simulink model "d_motor"  (Simulink 5.1)
settings: Solver=ode45  StartTime=0.0  StopTime=10.0  RelTol=1e-3
settings Model: Creator=fmilano  LastModifiedBy=fmilano  SignalLoggingName=logsout  BooleanDataType=on  RTWOptions="-aEnforceIntegerDowncast=1 -aFoldNonRolledExpr=1 -aInlineInvariantSignals=0 -aInlineParameters=0 -aLocalBlockOutputs=1 -aRollThreshold=5 -aZeroInternalMemoryAtStartup=1 -aZeroExternalMemoryAtStartup=1 -aInitFltsAndDblsToZero=0 -aForceBlockIOInitOptimize=0 -aGenerateReport=0 -aGenCodeOnly=0 -aRTWVerbose=1 -aIncludeHyperlinkInReport=0 -aLaunchReport=0 -aGenerateTraceInfo=0  -aForceParamTrailComments=0 -aGenerateComments=1 -aIgnoreCustomStorageClasses=1 -aIncHierarchyInIds=0 -aMaxRTWIdLen=31 -aShowEliminatedStatements=0 -aIncDataTypeInIds=0 -aInsertBlockDesc=0 -aIgnoreTestpoints=0 -aSimulinkBlockComments=1 -aInlinedPrmAccess=\"Literals\"  -aSuppressErrorStatus=0 -aModelReferenceCompliant=1 -aParenthesesLevel=\"Nominal\" -aModelStepFunctionPrototypeControlCompliant=0 -aPortableWordSizes=0 -aParMdlRefBuildCompliant=1 -aSupportNonInlinedSFcns=1 -aSupportContinuousTime=1 -aSupportComplex=1 -aSupportNonFinite=1 -aSupportAbsoluteTime=1 -aMultiwordLength=2048 -aTargetPreCompLibLocation=\"\" -aTargetLibSuffix=\"\" -aTargetFunctionLibrary=\"ANSI_C\" -aTargetFcnLib=\"ansi_tfl_tmw.mat\" -aMultiInstanceERTCode=0 -aLogVarNameModifier=\"rt_\" -aERTFirstTimeCompliant=0 -aIsPILTarget=0 -aCombineOutputUpdateFcns=0 -aGenerateASAP2=0 -aGenerateClassInterface=0 -aGenerateTestInterfaces=0 -aGenerateSampleERTMain=0 -aGenerateFullHeader=1 -aUtilityFuncGeneration=\"Auto\" -aIncludeFileDelimiter=\"Auto\" -aIncludeMdlTerminateFcn=1 -aPurelyIntegerCode=0 -aAutosarCompliant=0 -aERTCustomFileBanners=0 -aRTWCAPIStates=0 -aRTWCAPIParams=0 -aRTWCAPISignals=0 -aMatFileLogging=1 -aCompOptLevelCompliant=1 -aCPPClassGenCompliant=0 -aExtModeIntrfLevel=\"Level1\" -aExtModeMexFile=\"ext_comm\" -aExtModeTransport=0 -aExtModeStaticAllocSize=1000000 -aExtModeTesting=0 -aExtModeStaticAlloc=0 -aExtMode=0 -aERTMultiwordLength=256 -aERTMultiwordTypeDef=\"System defined\""

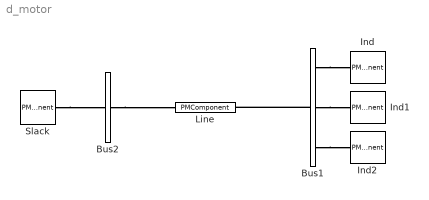
== system d_motor ==
  Bus1 : PMComponent  Tag=PSATblock  Description=Connection  PhysicalDomain=psatdomain  LeftPortType=p1  RightPortType=p1  LConnTagsString=__newl0  RConnTagsString=__newr0|__newr1|__newr2  mask(Bus){in=1, out=3, p2q=132, p3_4q=[1.00   0.00], p5q=1, p6q=1}
      mask prompts: in "Number of inputs:"; out "Number of outputs:"; p2q "Voltage Rating [kV]"; p3_4q "Voltage initial guess [p.u.   rad]"; p5q "Area number"; p6q "Region number"
      mask help: Bus block
      mask init:
      | fm_inout
      mask CallbackString: ||||fm_block|
      mask Display: plot([0 1 1 0 0],[0 0 1 1 0])
  Bus2 : PMComponent  Tag=PSATblock  Description=Connection  PhysicalDomain=psatdomain  LeftPortType=p1  RightPortType=p1  LConnTagsString=__newl0  RConnTagsString=__newr0  mask(Bus){in=1, out=1, p2q=132, p3_4q=[1.00   0.00], p5q=1, p6q=1}
      mask prompts: in "Number of inputs:"; out "Number of outputs:"; p2q "Voltage Rating [kV]"; p3_4q "Voltage initial guess [p.u.   rad]"; p5q "Area number"; p6q "Region number"
      mask help: Bus block
      mask init:
      | fm_inout
      mask CallbackString: ||||fm_block|
      mask Display: plot([0 1 1 0 0],[0 0 1 1 0])
  Ind : PMComponent  Tag=PSATblock  Description=Machines  PhysicalDomain=psatdomain  LeftPortType=p1  RightPortType=p1  LConnTagsString=__newl0  mask(Ind){p2_3_4q=[100   132   60], p5q=1, p6q=on, p7q=0.01, p8q=0.15, p9_10q=[0.05  0.15], p11_12q=[0.001  0.04], p13q=5.00, p14q=3.00, p15_16_17q=[0.5  0.00  0.00], p18q=0, p19q=off, p20q=on}
      mask prompts: p2_3_4q "Power, Voltage and Frequency Ratings [MVA, kV, Hz]"; p5q "Dynamic Order"; p6q "Start up"; p7q "Stator Resistance Rs [p.u.]"; p8q "Stator Reactance Xs [p.u.]"; p9_10q "First Cage Resitance Rr1 and Reactance  Xr1 [p.u. p.u.]"; p11_12q "Second Cage Resistance Rr2 and Reactance Xr2 [p.u.  p.u.]"; p13q "Magnetization Reactance Xm [p.u.]"; p14q "Inertia Constant Hm [kWs/kVA]"; p15_16_17q "Mechanical Torque coefficients [a, b, c] [p.u.  p.u.  p.u.]"; p18q "Start up time"; p19q "Allow working as brake"; p20q "Connected"
      mask help:
      | This block defines an asynchronous machine.
      |
      | Order 1:  mechanical equation
      | Order 3:  single cage
      | Order 5:  double cage
      mask init:
      | [x,y] = fm_draw('circle');
      | [xs,ys] = fm_draw('sinus');
      mask StyleString: edit,popup(1|3|5),checkbox,edit,edit,edit,edit,edit,edit,edit,edit,checkbox,checkbox
      mask CallbackString: |fm_block|||||||||||fm_block
      mask Display:
      | plot(x+1.4,y,0.12*xs+1,0.15*ys-0.6)
      | color('blue')
      | plot([1 1 1.4 1.8 1.8],[-0.05 0.7 0.4 0.7 -0.05])
  Ind1 : PMComponent  Tag=PSATblock  Description=Machines  PhysicalDomain=psatdomain  LeftPortType=p1  RightPortType=p1  LConnTagsString=__newl0  mask(Ind){p2_3_4q=[100   132   60], p5q=3, p6q=on, p7q=0.01, p8q=0.15, p9_10q=[0.05  0.15], p11_12q=[0.001  0.04], p13q=5.00, p14q=3.00, p15_16_17q=[0.25  0.00  0.00], p18q=1, p19q=off, p20q=on}
      mask prompts: p2_3_4q "Power, Voltage and Frequency Ratings [MVA, kV, Hz]"; p5q "Dynamic Order"; p6q "Start up"; p7q "Stator Resistance Rs [p.u.]"; p8q "Stator Reactance Xs [p.u.]"; p9_10q "First Cage Resitance Rr1 and Reactance  Xr1 [p.u. p.u.]"; p11_12q "Second Cage Resistance Rr2 and Reactance Xr2 [p.u.  p.u.]"; p13q "Magnetization Reactance Xm [p.u.]"; p14q "Inertia Constant Hm [kWs/kVA]"; p15_16_17q "Mechanical Torque coefficients [a, b, c] [p.u.  p.u.  p.u.]"; p18q "Start up time"; p19q "Allow working as brake"; p20q "Connected"
      mask help:
      | This block defines an asynchronous machine.
      |
      | Order 1:  mechanical equation
      | Order 3:  single cage
      | Order 5:  double cage
      mask init:
      | [x,y] = fm_draw('circle');
      | [xs,ys] = fm_draw('sinus');
      mask StyleString: edit,popup(1|3|5),checkbox,edit,edit,edit,edit,edit,edit,edit,edit,checkbox,checkbox
      mask CallbackString: |fm_block|||||||||||fm_block
      mask Display:
      | plot(x+1.4,y,0.12*xs+1,0.15*ys-0.6)
      | color('blue')
      | plot([1 1 1.4 1.8 1.8],[-0.05 0.7 0.4 0.7 -0.05])
  Ind2 : PMComponent  Tag=PSATblock  Description=Machines  PhysicalDomain=psatdomain  LeftPortType=p1  RightPortType=p1  LConnTagsString=__newl0  mask(Ind){p2_3_4q=[100   132   60], p5q=5, p6q=off, p7q=0.01, p8q=0.15, p9_10q=[0.05  0.15], p11_12q=[0.001  0.04], p13q=5.00, p14q=3.00, p15_16_17q=[0.13  0.02  0.024], p18q=1, p19q=off, p20q=on}
      mask prompts: p2_3_4q "Power, Voltage and Frequency Ratings [MVA, kV, Hz]"; p5q "Dynamic Order"; p6q "Start up"; p7q "Stator Resistance Rs [p.u.]"; p8q "Stator Reactance Xs [p.u.]"; p9_10q "First Cage Resitance Rr1 and Reactance  Xr1 [p.u. p.u.]"; p11_12q "Second Cage Resistance Rr2 and Reactance Xr2 [p.u.  p.u.]"; p13q "Magnetization Reactance Xm [p.u.]"; p14q "Inertia Constant Hm [kWs/kVA]"; p15_16_17q "Mechanical Torque coefficients [a, b, c] [p.u.  p.u.  p.u.]"; p18q "Start up time"; p19q "Allow working as brake"; p20q "Connected"
      mask help:
      | This block defines an asynchronous machine.
      |
      | Order 1:  mechanical equation
      | Order 3:  single cage
      | Order 5:  double cage
      mask init:
      | [x,y] = fm_draw('circle');
      | [xs,ys] = fm_draw('sinus');
      mask StyleString: edit,popup(1|3|5),checkbox,edit,edit,edit,edit,edit,edit,edit,edit,checkbox,checkbox
      mask CallbackString: |fm_block|||||||||||fm_block
      mask Display:
      | plot(x+1.4,y,0.12*xs+1,0.15*ys-0.6)
      | color('blue')
      | plot([1 1 1.4 1.8 1.8],[-0.05 0.7 0.4 0.7 -0.05])
  Line : PMComponent  Tag=PSATblock  Description=Power Flow  PhysicalDomain=psatdomain  LeftPortType=p1  RightPortType=p1  LConnTagsString=__newl0  RConnTagsString=__newr0  mask(Line){p3_4_5q=[100  132  60], p6q=0, p8q=0.01, p9q=0.10, p10q=1e-3, p13_14_15q=[0.0  0.0  0.0], p16q=on}
      mask prompts: p3_4_5q "Power, Voltage and Frequency Ratings [MVA, kV, Hz]"; p6q "Length of line [km] (0 for p.u. parameters)"; p8q "Resistance [p.u. (Ohms/km)]"; p9q "Reactance [p.u. (H/km)]"; p10q "Susceptance [p.u. (F/km)]"; p13_14_15q "Imax, Pmax and Smax [p.u., p.u., p.u.]"; p16q "Connected"
      mask help: This block defines a pi model for a tree phase line.
      mask init:
      | [xp,yp] = fm_draw('pi');
      mask CallbackString: ||||||fm_block
      mask Display:
      | plot([-1  1  1 -1 -1],[-0.2 -0.2 0.2 0.2 -0.2])
      | color('blue')
      | plot(0.35*xp,0.2*yp)
  Slack : PMComponent  Tag=PSATblock  Description=Power Flow  PhysicalDomain=psatdomain  LeftPortType=p1  RightPortType=p1  RConnTagsString=__newr0  mask(SW){p2_3q=[100  132], p4q=1.05, p5q=0.00, p6_7q=[1.5  -1.5], p8_9q=[1.1  0.9], p10q=0.80, p11q=1, p12q=on, p13q=on}
      mask prompts: p2_3q "Power and Voltage Ratings [MVA, kV]"; p4q "Voltage Magnitude [p.u.]"; p5q "Reference Phase Angle [rad]"; p6_7q "Qmax and Qmin [p.u.  p.u.]"; p8_9q "Vmax and Vmin  [p.u.  p.u.]"; p10q "Active Power Guess [p.u.]"; p11q "Loss Participation Factor"; p12q "Reference bus"; p13q "Connected"
      mask help:
      | This block defines a V-theta bus:
      |
      | V = V_des
      | theta = theta_des
      mask init:
      | [x,y] = fm_draw('circle');
      | [xt,yt] = fm_draw('theta');
      mask CallbackString: |||||||fm_block|fm_block
      mask Display: plot([0 1 1 0 0],[0 0 1 1 0]), color('blue'), plot([0 1],[0 1],[0 1],[1 0],[0.5 1 0.5 0 0.5],[0 0.5 1 0.5 0])
  connections:
  Slack/RConn1 -- Bus2/LConn1
  Bus2/RConn1 -- Line/LConn1
  Bus1/LConn1 -- Line/RConn1
  Bus1/RConn1 -- Ind/LConn1
  Bus1/RConn2 -- Ind1/LConn1
  Bus1/RConn3 -- Ind2/LConn1
